simulink model "kaihuan"  (R2023b)
settings: Solver=VariableStepAuto  StartTime=0.0  StopTime=0.02  RelTol=1e-3
libraries: spsMosfetLib x8, spsSeriesRLCBranchLib x5, spsMultimeterLib x2, simulink x2, spsDCVoltageSourceLib x1, spsLinearTransformerLib x1, spsVoltageMeasurementLib x1, sps_lib x1
settings Model: Creator=ASUS  LastModifiedBy=ASUS

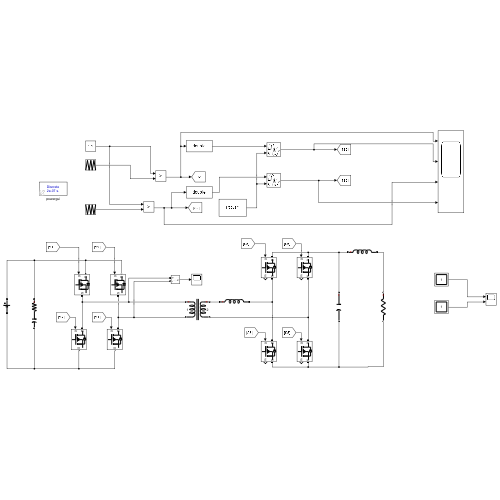
[thumbnail: Simulink's stored preview of the top-level diagram]
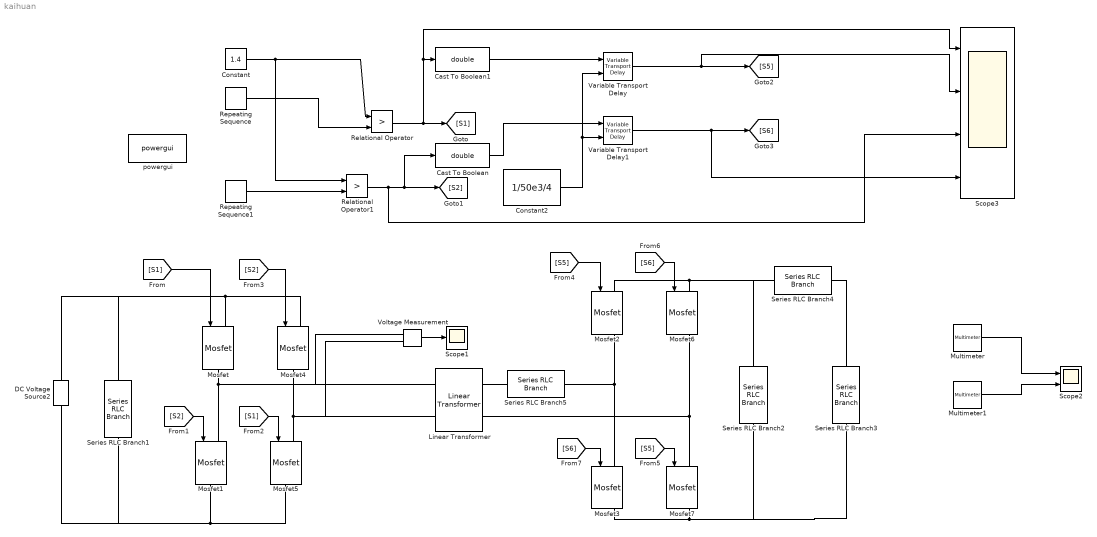
== system kaihuan ==
  Cast To Boolean : DataTypeConversion  OutDataTypeStr=double  SaturateOnIntegerOverflow=off  RndMeth=Floor
  Cast To Boolean1 : DataTypeConversion  OutDataTypeStr=double  SaturateOnIntegerOverflow=off  RndMeth=Floor
  Constant : Constant  Value=1.4
  Constant2 : Constant  Value=1/50e3/4
  DC Voltage Source2 : spsDCVoltageSourceLib/DC Voltage Source  Amplitude=48  Measurements=None
  Linear Transformer : spsLinearTransformerLib/Linear Transformer  UNITS=pu  NominalPower=[ 1e3 50e3 ]  winding1=[92 0.000002 0.079997]  winding2=[410 0.00002 0.079999]  ThreeWindings=off  winding3=[3.15e+05 4e-10 1.3333e-05]  RmLm=[500 500]  Measurements=None  DataType=off
  Mosfet{,1,4..5} (4 alike) : spsMosfetLib/Mosfet  Ron=0.1  Lon=0  Rd=0.01  Vfd=0  IC=0  Rs=1e5  Cs=inf  Measurements=off
  Mosfet{2..3,6..7} (4 alike) : spsMosfetLib/Mosfet  Ron=0.1  Lon=0  Rd=0.01  Vfd=0  IC=0  Rs=1e5  Cs=inf  Measurements=on
  Multimeter : spsMultimeterLib/Multimeter  L=2  sel=1  yselected={}  Gain=1  OutputType=Complex  PlotAtSimulationStop=off  PhasorSimulation=off
  Multimeter1 : spsMultimeterLib/Multimeter  L=2  sel=2  yselected={}  Gain=1  OutputType=Complex  PlotAtSimulationStop=off  PhasorSimulation=off
  Relational Operator : RelationalOperator  Operator=>  OutDataTypeStr=boolean  RndMeth=Simplest  InputSameDT=off
  Relational Operator1 : RelationalOperator  Operator=>  OutDataTypeStr=boolean  RndMeth=Simplest  InputSameDT=off
  Repeating Sequence : simulink/Sources/Repeating Sequence  rep_seq_t=[0 1/50e3/2 1/50e3]  rep_seq_y=[0 3 0]
  Repeating Sequence1 : simulink/Sources/Repeating Sequence  rep_seq_t=[0 1/50e3/2 1/50e3]  rep_seq_y=[3 0 3]
  Scope1 : Scope
  Scope2 : Scope  NumInputPorts=2
  Scope3 : Scope  NumInputPorts=4
  Series RLC Branch1 : spsSeriesRLCBranchLib/Series RLC Branch  LConnTagsString=__new0  RConnTagsString=__new0  BranchType=RC  Resistance=0.0001  Inductance=1e-3  SetiL0=off  InitialCurrent=0  Capacitance=51e-6  Setx0=off  InitialVoltage=0  Measurements=None
  Series RLC Branch2 : spsSeriesRLCBranchLib/Series RLC Branch  LConnTagsString=__new0  RConnTagsString=__new0  BranchType=C  Resistance=0.000001  Inductance=1e-3  SetiL0=off  InitialCurrent=0  Capacitance=2e-6  Setx0=off  InitialVoltage=0  Measurements=None
  Series RLC Branch3 : spsSeriesRLCBranchLib/Series RLC Branch  LConnTagsString=__new0  RConnTagsString=__new0  BranchType=R  Resistance=160  Inductance=1e-3  SetiL0=off  InitialCurrent=0  Capacitance=1e-6  Setx0=off  InitialVoltage=0  Measurements=Branch voltage and current
  Series RLC Branch4 : spsSeriesRLCBranchLib/Series RLC Branch  LConnTagsString=__new0  RConnTagsString=__new0  BranchType=L  Resistance=1  Inductance=600e-6  SetiL0=off  InitialCurrent=0  Capacitance=1e-6  Setx0=off  InitialVoltage=0  Measurements=None
  Series RLC Branch5 : spsSeriesRLCBranchLib/Series RLC Branch  LConnTagsString=__new0  RConnTagsString=__new0  BranchType=L  Resistance=1  Inductance=98e-6  SetiL0=off  InitialCurrent=0  Capacitance=1e-6  Setx0=off  InitialVoltage=0  Measurements=None
  Variable Transport Delay : VariableTransportDelay  VariableDelayType=Variable transport delay  MaximumDelay=10
  Variable Transport Delay1 : VariableTransportDelay  VariableDelayType=Variable transport delay  MaximumDelay=10
  Voltage Measurement : spsVoltageMeasurementLib/Voltage Measurement  PhasorSimulation=off  OutputType=Complex  PSBequivalent=0
  powergui : sps_lib/powergui  Priority=1  SimulationMode=Discrete  SampleTime=2e-07  frequency=60  Iterations=50  frequencyindice=0  Pbase=100e6  ErrMax=1e-4  UnitsV=kV  UnitsW=MW  buscounter=0  FunctionMessages=off  echomessages=off  EnableUseOfTLC=off  CurrentSourceSwitches=off  DisableSnubberDevices=off  DisableRonSwitches=off  DisableVfSwitches=off  DisplayEquations=off  AutomaticDiscreteSolvers=off  SolverType=Tustin/Backward Euler (TBE)  Interpol=off  ExternalGateDelay=off  methode=off  Ts=100  x0status=blocks  SPID=on  SwTol=0  HookPort=off  NonlinearTolerance=1e-4  nMaxIteration=100  ContinueOnMaxIteration=off  RestoreLinks=warning  ResistiveCurrentMeasurement=off  Frange=[0:2:500]  Ylog=off  Xlog=on  ShowGrid=off  save=off  variable=ZData  structure=0  ZoomFFT=off  StartTime=0.0  cycles=1  DisplayStyle=1  fundamental=60  FreqAxis=off  MaxFrequency=1000  frequencyindicesteady=1  RmsSteady=1  display=off
  wires:
  Constant/1 -> Relational Operator1/1, Relational Operator/1
  Repeating Sequence/1 -> Relational Operator/2
  Repeating Sequence1/1 -> Relational Operator1/2
  [S1] -> Mosfet/1
  [S2] -> Mosfet1/1
  [S1] -> Mosfet5/1
  [S2] -> Mosfet4/1
  Voltage Measurement/1 -> Scope1/1
  Relational Operator/1 -> Scope3/1, Cast To Boolean1/1, [S1]
  [S6] -> Mosfet6/1
  [S6] -> Mosfet3/1
  [S5] -> Mosfet2/1
  [S5] -> Mosfet7/1
  Variable Transport Delay1/1 -> Scope3/4, [S6]
  Variable Transport Delay/1 -> Scope3/2, [S5]
  Cast To Boolean1/1 -> Variable Transport Delay/1
  Cast To Boolean/1 -> Variable Transport Delay1/1
  Relational Operator1/1 -> Scope3/3, Cast To Boolean/1, [S2]
  Constant2/1 -> Variable Transport Delay/2, Variable Transport Delay1/2
  Multimeter/1 -> Scope2/1
  Multimeter1/1 -> Scope2/2
  connections:
  Mosfet/LConn1 -- DC Voltage Source2/RConn1 -- Series RLC Branch1/LConn1 -- Mosfet4/LConn1
  Mosfet5/RConn1 -- DC Voltage Source2/LConn1 -- Series RLC Branch1/RConn1 -- Mosfet1/RConn1
  Mosfet5/LConn1 -- Linear Transformer/LConn2 -- Voltage Measurement/LConn2 -- Mosfet4/RConn1
  Mosfet1/LConn1 -- Linear Transformer/LConn1 -- Voltage Measurement/LConn1 -- Mosfet/RConn1
  Mosfet3/LConn1 -- Series RLC Branch5/RConn1 -- Mosfet2/RConn1
  Mosfet7/LConn1 -- Linear Transformer/RConn2 -- Mosfet6/RConn1
  Mosfet7/RConn1 -- Series RLC Branch3/RConn1 -- Series RLC Branch2/RConn1 -- Mosfet3/RConn1
  Mosfet6/LConn1 -- Series RLC Branch4/LConn1 -- Series RLC Branch2/LConn1 -- Mosfet2/LConn1
  Linear Transformer/RConn1 -- Series RLC Branch5/LConn1
  Series RLC Branch3/LConn1 -- Series RLC Branch4/RConn1
